simulink model "lss_online"  (R2022b)
settings: Solver=FixedStepAuto  StartTime=0.0  StopTime=Inf  FixedStep=0.001  RelTol=1e-3  EnableMultiTasking=on
InitFcn:
  | clear mex
model workspace (MAT data in the model file):
  worldsim_instance : object (value not decoded)
values from neighbouring files (symbols this model uses):
  ADAS_Control_Mode = 1    [LSS_parameters.m]    (also in lss_ini_param.sldd = 1.0)
  AP_Transition_Rate = 0.5    [LSS_parameters.m]    (also in lss_ini_param.sldd = 0.8)
  butter_a = 1.0 -1.9911142922016536 0.99115359586893548    [lss_ini_param.sldd]
  butter_a_lka_out = 1.0 -1.5610180758007179 0.641351538057563    [lss_ini_param.sldd]
  butter_b = 9.825916820482009E-6 1.9651833640964018E-5 9.825916820482009E-6    [lss_ini_param.sldd]
  butter_b_lka_out = 0.020083365564211246 0.040166731128422492 0.020083365564211246    [lss_ini_param.sldd]
  index_variant_approaching_speed = 3.0    [lss_ini_param.sldd]
  LDW_Activity_Flag = 1    [LSS_parameters.m]    (also in lss_ini_param.sldd = 1.0)
  LDW_Freq_Hz = Sensor_Freq_worldsim    [LSS_parameters.m]    (also in lss_ini_param.sldd = 50.0)
  LDW_LaneGap_dydt_Warning = 50    [LSS_parameters.m]    (also in lss_ini_param.sldd = 50.0)
  LDW_LaneGap_Warning = [0.5 0.25]    [LSS_parameters.m]    (also in lss_ini_param.sldd = 0.5 0.25)
  LDW_Min_Speed = 60    [LSS_parameters.m]    (also in lss_ini_param.sldd = 60.0)
  LDW_Steer_Vibration_Amplitude = 5    [LSS_parameters.m]    (also in lss_ini_param.sldd = 5.0)
  LDW_Steer_Vibration_Freq = 25    [LSS_parameters.m]    (also in lss_ini_param.sldd = 25.0)
  LKA_Activity_Flag = 1    [LSS_parameters.m]    (also in lss_ini_param.sldd = 1.0)
  LKA_D = [0.2 0.3]    [LSS_parameters.m]    (also in lss_ini_param.sldd = 0.2 0.3)
  LKA_Dyn_Rate_Limiter_Gain = 0.1    [LSS_parameters.m]    (also in lss_ini_param.sldd)
  LKA_Dyn_Rate_Limiter_Power = 10    [LSS_parameters.m]    (also in lss_ini_param.sldd = 10.0)
  LKA_Error_dydt_Off = 1    [LSS_parameters.m]    (also in lss_ini_param.sldd = 1.0)
  LKA_Error_Max = 3    [LSS_parameters.m]    (also in lss_ini_param.sldd = 3.0)
  LKA_Error_Off = 0.5    [LSS_parameters.m]    (also in lss_ini_param.sldd)
  LKA_Freq_Hz = Sensor_Freq_worldsim    [LSS_parameters.m]    (also in lss_ini_param.sldd = 50.0)
  LKA_I = [0.025 0.05]    [LSS_parameters.m]    (also in lss_ini_param.sldd = 0.025 0.05)
  LKA_Lane_Gap_Activate = [0.25 0.125]    [LSS_parameters.m]    (also in lss_ini_param.sldd = -0.05 0.125)
  LKA_Lane_Gap_dydt_Activate = 50    [LSS_parameters.m]    (also in lss_ini_param.sldd = 50.0)
  LKA_Min_Speed = 60    [LSS_parameters.m]    (also in lss_ini_param.mat = 50; lss_ini_param.sldd = 50.0)
  LKA_On_Display_Freq = 5    [LSS_parameters.m]    (also in lss_ini_param.sldd = 5.0)
  LKA_P = [0.1 0.2]    [LSS_parameters.m]    (also in lss_ini_param.sldd = 0.1 0.2)
  LKA_Steer_Rate_Max_radps = 1    [LSS_parameters.m]    (also in lss_ini_param.sldd = 1.0)
  radar_source = 2    [LSS_parameters.m]    (also in lss_ini_param.sldd = 2.0)
  Sensor_Freq_worldsim = 50    [launcher.m]    (also in lss_ini_param.sldd = 50.0)
  target_speed = 72    [LSS_parameters.m]    (also in launcher.m = initCond.initialVelocity * 3.6)
  variant_approaching_speed = v_lat    [launcher.m]    (also in lss_ini_param.sldd = 0.2 0.3 0.4 0.5 0.6)
  vehicle_width = 1.86    [LSS_parameters.m]    (also in lss_ini_param.sldd = 2.05)
libraries: simulink x41, simwbSfunlib x40, slpidlib x3, viworldsim_lib x3
(part 2 of 2)

== system lss_online/INPUT/simple_cruise_control ==
  note: This is used to mantaint the target speed until controller action
  Cast To Double : DataTypeConversion  OutDataTypeStr=double  SaturateOnIntegerOverflow=off  RndMeth=Floor
  Compare To Constant4 : simulink/Logic and Bit Operations/Compare To Constant  relop===  const=0  OutDataTypeStr=boolean
  Compare To Constant5 : simulink/Logic and Bit Operations/Compare To Constant  relop===  const=0  OutDataTypeStr=boolean
  Constant : Constant  Value=0
  PID Controller : slpidlib/PID Controller  Controller=PI  Form=Parallel  TimeDomain=Discrete-time  UseExternalTs=off  SampleTime=-1  IntegratorMethod=Forward Euler  FilterMethod=Forward Euler  ControllerParametersSource=internal  P=40  I=10  UseKiTs=off  D=0  N=100  UseFilter=on  TunerSelectOption=Transfer Function Based (PID Tuner App)  InitialConditionSource=internal  InitialConditionForIntegrator=0  InitialConditionForFilter=0  DifferentiatorICPrevScaledInput=0  ExternalReset=none  TrackingMode=off  Kt=1  LimitOutput=on  SatLimitsSource=internal  UpperSaturationLimit=100  LowerSaturationLimit=0  LinearizeAsGain=on  AntiWindupMode=none  Kb=1  LimitIntegrator=off  UpperIntegratorSaturationLimit=inf  LowerIntegratorSaturationLimit=-inf  POutMin=[]  POutMax=[]  IOutMin=[]  IOutMax=[]  DOutMin=[]  DOutMax=[]  NOutMin=[]  NOutMax=[]  SumOutMin=[]  SumOutMax=[]  SaturationOutMin=[]  SaturationOutMax=[]  PParamMin=[]  PParamMax=[]  IParamMin=[]  IParamMax=[]  DParamMin=[]  DParamMax=[]  NParamMin=[]  NParamMax=[]  KbParamMin=[]  KbParamMax=[]  KtParamMin=[]  KtParamMax=[]  KbOutMin=[]  KbOutMax=[]  KtOutMin=[]  KtOutMax=[]  IntegratorOutMin=[]  IntegratorOutMax=[]  FilterOutMin=[]  FilterOutMax=[]  SumI1OutMin=[]  SumI1OutMax=[]  SumI2OutMin=[]  SumI2OutMax=[]  SumI3OutMin=[]  SumI3OutMax=[]  SumI4OutMin=[]  SumI4OutMax=[]  SumDOutMin=[]  SumDOutMax=[]  DifferentiatorOutMin=[]  DifferentiatorOutMax=[]  FilterDiffOutCoefMin=[]  FilterDiffOutCoefMax=[]  ReciprocalOutMin=[]  ReciprocalOutMax=[]  SumDenOutMin=[]  SumDenOutMax=[]  SumNumOutMin=[]  SumNumOutMax=[]  DivideOutMin=[]  DivideOutMax=[]  UdiffTsProdOutMin=[]  UdiffTsProdOutMax=[]  NTsProdOutMin=[]  NTsProdOutMax=[]  UintegralTsProdOutMin=[]  UintegralTsProdOutMax=[]  UngainTsProdOutMin=[]  UngainTsProdOutMax=[]  ClampingZeroOutDataTypeStr=Inherit: Inherit via back propagation  ClampingZeroOutMin=[]  ClampingZeroOutMax=[]  FilterDenConstantOutDataTypeStr=Inherit: Inherit via back propagation  FilterDenConstantOutMin=[]  FilterDenConstantOutMax=[]  PCopyOutDataTypeStr=Inherit: Inherit via back propagation  PCopyOutMin=[]  PCopyOutMax=[]  NCopyOutDataTypeStr=Inherit: Inherit via back propagation  NCopyOutMin=[]  NCopyOutMax=[]  IntegratorContinuousStateAttributes=''  IntegratorStateMustResolveToSignalObject=off  IntegratorRTWStateStorageClass=Auto  FilterContinuousStateAttributes=''  FilterStateMustResolveToSignalObject=off  FilterRTWStateStorageClass=Auto  ParallelPVariant=InternalParameters  IdealPVariant=Disabled  IVariant=InternalParameters  DVariant=Disabled  IntegratorVariant=Discrete  SatVariant=Enabled  AWVariant=Passthrough  PCopyVariant=Disabled  TRVariant=Disabled  FdbkBlocksVariant=Forward  IdealPFdbkVariant=Disabled  SatFdbkVariant=Disabled  DerivativeFilterVariant=Disabled  NVariant=Disabled  NCopyVariant=Disabled_SignalSpec  FilterICVariant=Disabled  IntegratorICVariant=InternalICs  ExternalResetVariant=Disabled  TRSumVariant=Passthrough  SumFdbkVariant=Disabled  SumVariant=Sum_PI  TsampFilterVariant=InternalTs  TsampNgainVariant=Passthrough  TsampIntegralVariant=Passthrough  ExternalSaturationOutDataTypeStr=Inherit: Same as second input
  Product : Product
  Sum : Sum  Inputs=+-
  target_speed_ : Constant  Value=target_speed
  tag scope: CC_clutch_demand=global, CC_throttle_demand=global
  wires:
  target_speed_/1 -> Sum/1
  Sum/1 -> PID Controller/1
  [Vehicle_Speed] -> Sum/2
  PID Controller/1 -> Product/1  "throttle"
  Product/1 -> Compare To Constant4/1, [CC_throttle_demand]
  Compare To Constant5/1 -> Product/2
  [AEB_Output_Brake] -> Compare To Constant5/1
  Compare To Constant4/1 -> Cast To Double/1
  Cast To Double/1 -> [CC_clutch_demand]
  Constant/1 -> [AEB_Output_Brake]

== system lss_online/LDW/LDW_LaneGap_Warning1 ==
  In1 : Inport
  ADAS_Control_Mode : Constant  Value=ADAS_Control_Mode
  LDW_LaneGap_Warning : Constant  Value=LDW_LaneGap_Warning(1)
  LDW_LaneGap_Warning1 : Constant  Value=LDW_LaneGap_Warning(2)  VectorParams1D=off
  Multiport Switch : MultiPortSwitch  Inputs=2  DataPortForDefault=Additional data port  DiagnosticForDefault=None  SaturateOnIntegerOverflow=off  InputSameDT=off
  Relational Operator : RelationalOperator  Operator=<  OutDataTypeStr=boolean  InputSameDT=off
  Out1 : Outport  VectorParamsAs1DForOutWhenUnconnected=off
  wires:
  ADAS_Control_Mode/1 -> Multiport Switch/1
  Multiport Switch/1 -> Relational Operator/2
  Relational Operator/1 -> Out1/1
  In1/1 -> Relational Operator/1
  LDW_LaneGap_Warning/1 -> Multiport Switch/4, Multiport Switch/2
  LDW_LaneGap_Warning1/1 -> Multiport Switch/3

== system lss_online/LKA/Discrete PID Controller ==
  In1 : Inport
  In2 : Inport  Port=2
  ADAS_Control_Mode : Constant  Value=ADAS_Control_Mode
  Demux : Demux  Outputs=3
  Discrete PID Controller : slpidlib/PID Controller  Controller=PID  Form=Parallel  TimeDomain=Discrete-time  UseExternalTs=off  SampleTime=1/LKA_Freq_Hz  IntegratorMethod=Forward Euler  FilterMethod=Forward Euler  ControllerParametersSource=external  P=LKA_P  I=LKA_I  UseKiTs=off  D=LKA_D  N=100  UseFilter=off  TunerSelectOption=Transfer Function Based (PID Tuner App)  InitialConditionSource=internal  InitialConditionForIntegrator=0  InitialConditionForFilter=0  DifferentiatorICPrevScaledInput=0  ExternalReset=either  TrackingMode=off  Kt=1  LimitOutput=off  SatLimitsSource=internal  UpperSaturationLimit=inf  LowerSaturationLimit=-inf  LinearizeAsGain=off  AntiWindupMode=clamping  Kb=1  LimitIntegrator=off  UpperIntegratorSaturationLimit=inf  LowerIntegratorSaturationLimit=-inf  POutMin=[]  POutMax=[]  IOutMin=[]  IOutMax=[]  DOutMin=[]  DOutMax=[]  NOutMin=[]  NOutMax=[]  SumOutMin=[]  SumOutMax=[]  SaturationOutMin=[]  SaturationOutMax=[]  PParamMin=[]  PParamMax=[]  IParamMin=[]  IParamMax=[]  DParamMin=[]  DParamMax=[]  NParamMin=[]  NParamMax=[]  KbParamMin=[]  KbParamMax=[]  KtParamMin=[]  KtParamMax=[]  KbOutMin=[]  KbOutMax=[]  KtOutMin=[]  KtOutMax=[]  IntegratorOutMin=[]  IntegratorOutMax=[]  FilterOutMin=[]  FilterOutMax=[]  SumI1OutMin=[]  SumI1OutMax=[]  SumI2OutMin=[]  SumI2OutMax=[]  SumI3OutMin=[]  SumI3OutMax=[]  SumI4OutMin=[]  SumI4OutMax=[]  SumDOutMin=[]  SumDOutMax=[]  DifferentiatorOutMin=[]  DifferentiatorOutMax=[]  FilterDiffOutCoefMin=[]  FilterDiffOutCoefMax=[]  ReciprocalOutMin=[]  ReciprocalOutMax=[]  SumDenOutMin=[]  SumDenOutMax=[]  SumNumOutMin=[]  SumNumOutMax=[]  DivideOutMin=[]  DivideOutMax=[]  UdiffTsProdOutMin=[]  UdiffTsProdOutMax=[]  NTsProdOutMin=[]  NTsProdOutMax=[]  UintegralTsProdOutMin=[]  UintegralTsProdOutMax=[]  UngainTsProdOutMin=[]  UngainTsProdOutMax=[]  ClampingZeroOutDataTypeStr=Inherit: Inherit via back propagation  ClampingZeroOutMin=[]  ClampingZeroOutMax=[]  FilterDenConstantOutDataTypeStr=Inherit: Inherit via back propagation  FilterDenConstantOutMin=[]  FilterDenConstantOutMax=[]  PCopyOutDataTypeStr=Inherit: Inherit via back propagation  PCopyOutMin=[]  PCopyOutMax=[]  NCopyOutDataTypeStr=Inherit: Inherit via back propagation  NCopyOutMin=[]  NCopyOutMax=[]  IntegratorContinuousStateAttributes=''  IntegratorStateMustResolveToSignalObject=off  IntegratorRTWStateStorageClass=Auto  FilterContinuousStateAttributes=''  FilterStateMustResolveToSignalObject=off  FilterRTWStateStorageClass=Auto  ParallelPVariant=ExternalParameters  IdealPVariant=Disabled  IVariant=ExternalParameters  DVariant=ExternalParameters  IntegratorVariant=Discrete  SatVariant=Disabled  AWVariant=Passthrough  PCopyVariant=Disabled  TRVariant=Disabled  FdbkBlocksVariant=Forward  IdealPFdbkVariant=Disabled  SatFdbkVariant=Disabled  DerivativeFilterVariant=Differentiator  NVariant=Passthrough  NCopyVariant=Disabled_SignalSpec  FilterICVariant=InternalICsDifferentiator  IntegratorICVariant=InternalICs  ExternalResetVariant=ExternalReset  TRSumVariant=Passthrough  SumFdbkVariant=Disabled  SumVariant=Sum_PID  TsampFilterVariant=InternalTs  TsampNgainVariant=Passthrough  TsampIntegralVariant=Passthrough  ExternalSaturationOutDataTypeStr=Inherit: Same as second input
  LKA_D(1) : Constant  Value=LKA_D(1)
  LKA_D(1)1 : Constant  Value=LKA_D(2)
  LKA_I(1) : Constant  Value=LKA_I(1)
  LKA_I(1)1 : Constant  Value=LKA_I(2)
  LKA_P(1) : Constant  Value=LKA_P(1)
  LKA_P(1)1 : Constant  Value=LKA_P(2)
  Multiport Switch : MultiPortSwitch  Inputs=2  DataPortForDefault=Additional data port  DiagnosticForDefault=None  SaturateOnIntegerOverflow=off  InputSameDT=off
  Mux : Mux  Inputs=3
  Mux1 : Mux  Inputs=3
  Out1 : Outport  VectorParamsAs1DForOutWhenUnconnected=off
  wires:
  In1/1 -> Discrete PID Controller/1
  In2/1 -> Discrete PID Controller/5
  Discrete PID Controller/1 -> Out1/1
  LKA_P(1)/1 -> Mux/1
  ADAS_Control_Mode/1 -> Multiport Switch/1
  Demux/2 -> Discrete PID Controller/3
  Demux/3 -> Discrete PID Controller/4
  Demux/1 -> Discrete PID Controller/2
  Mux1/1 -> Multiport Switch/3
  Mux/1 -> Multiport Switch/4, Multiport Switch/2
  LKA_I(1)/1 -> Mux/2
  LKA_D(1)/1 -> Mux/3
  LKA_P(1)1/1 -> Mux1/1
  LKA_I(1)1/1 -> Mux1/2
  LKA_D(1)1/1 -> Mux1/3
  Multiport Switch/1 -> Demux/1

== system lss_online/LKA/LKA_Lane_Gap_Activate ==
  In1 : Inport
  ADAS_Control_Mode : Constant  Value=ADAS_Control_Mode
  LKA_Lane_Gap_Activate : Constant  Value=LKA_Lane_Gap_Activate(1)
  LKA_Lane_Gap_Activate2 : Constant  Value=LKA_Lane_Gap_Activate(2)  VectorParams1D=off
  Multiport Switch : MultiPortSwitch  Inputs=2  DataPortForDefault=Additional data port  DiagnosticForDefault=None  SaturateOnIntegerOverflow=off  InputSameDT=off
  Relational Operator : RelationalOperator  Operator=<  OutDataTypeStr=boolean  InputSameDT=off
  Out1 : Outport  VectorParamsAs1DForOutWhenUnconnected=off
  wires:
  ADAS_Control_Mode/1 -> Multiport Switch/1
  Multiport Switch/1 -> Relational Operator/2
  Relational Operator/1 -> Out1/1
  In1/1 -> Relational Operator/1
  LKA_Lane_Gap_Activate/1 -> Multiport Switch/4, Multiport Switch/2
  LKA_Lane_Gap_Activate2/1 -> Multiport Switch/3

== system lss_online/LKA/Subsystem ==
  Clock : Inport
  Input_Signal : Inport  Port=2
  Delay : Delay  DelayLength=1000/LKA_Freq_Hz  InitialCondition=-1/LKA_Freq_Hz
  Delay1 : Delay  DelayLength=1000/LKA_Freq_Hz
  Delay2 : Delay  DelayLength=1000/LKA_Freq_Hz
  Lookup Table Dynamic : simulink/Lookup Tables/Lookup Table Dynamic  LookUpMeth=Interpolation-Use End Values  OutDataType=fixdt('double')  OutScaling=[]  OutputDataTypeScalingMode=Specify via dialog  OutDataTypeStr=fixdt('double')  DoSatur=off
  Vector Concatenate : Concatenate
  Vector Concatenate1 : Concatenate
  Zero-Order Hold1 : ZeroOrderHold  SampleTime=1/LKA_Freq_Hz
  Zero-Order Hold2 : ZeroOrderHold  SampleTime=1/LKA_Freq_Hz
  Zero-Order Hold3 : ZeroOrderHold  SampleTime=1e-3
  Zero-Order Hold4 : ZeroOrderHold  SampleTime=1e-3
  1kHz_Interpolation : Outport  VectorParamsAs1DForOutWhenUnconnected=off
  wires:
  Input_Signal/1 -> Zero-Order Hold1/1
  Zero-Order Hold1/1 -> Zero-Order Hold4/1
  Zero-Order Hold3/1 -> Delay/1, Vector Concatenate/2
  Zero-Order Hold2/1 -> Zero-Order Hold3/1
  Delay/1 -> Vector Concatenate/1
  Delay1/1 -> Lookup Table Dynamic/1
  Delay2/1 -> Vector Concatenate1/1
  Zero-Order Hold4/1 -> Delay2/1, Vector Concatenate1/2
  Vector Concatenate1/1 -> Lookup Table Dynamic/3
  Vector Concatenate/1 -> Lookup Table Dynamic/2
  Clock/1 -> Delay1/1, Zero-Order Hold2/1
  Lookup Table Dynamic/1 -> 1kHz_Interpolation/1

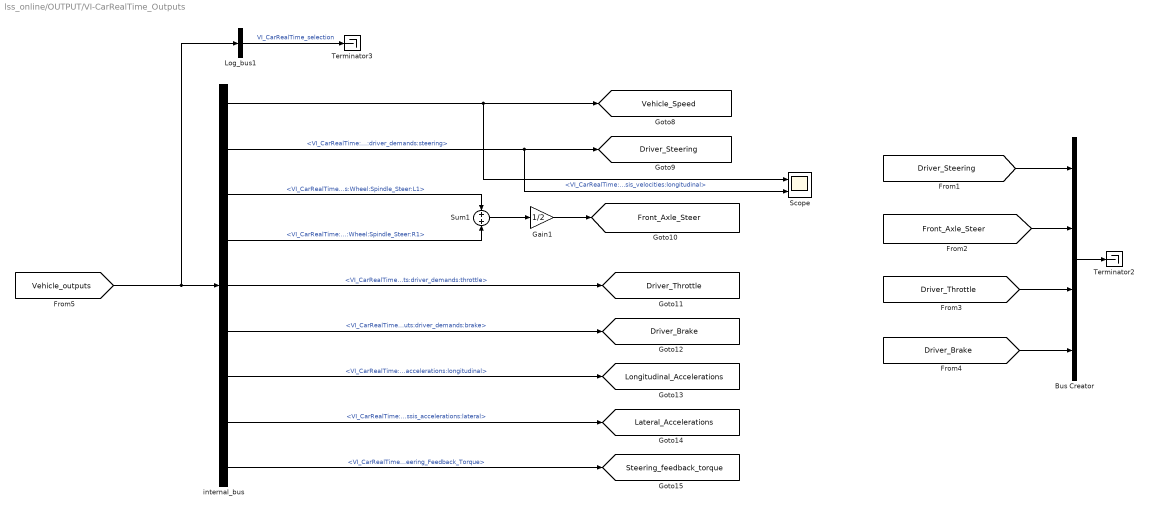
== system lss_online/OUTPUT/VI-CarRealTime_Outputs ==
  Bus Creator : BusCreator  Inputs=4
  Gain1 : Gain  Gain=1/2
  Log_bus1 : BusSelector  OutputSignals=VI_CarRealTime:Outputs:chassis_velocities:longitudinal,VI_CarRealTime:Outputs:driver_demands:steering,VI_CarRealTime:Outputs:Wheel:Spindle_Steer:L1,VI_CarRealTime:Outputs:Wheel:Spindle_Steer:R1,VI_CarRealTime:Outputs:driver_demands:throttle,VI_CarRealTime:Outputs:driver_demands:brake,VI_CarRealTime:Outputs:chassis_accelerations:longitudinal,VI_CarRealTime:Outputs:chassis_accelerations:lateral,VI_CarRealTime:Outputs:Steering_System:DriveSim_Steering_Feedback_Torque  OutputAsBus=on
  Scope : Scope  NumInputPorts=2
  Sum1 : Sum
  Terminator2 : Terminator
  Terminator3 : Terminator
  internal_bus : BusSelector  OutputSignals=VI_CarRealTime:Outputs:chassis_velocities:longitudinal,VI_CarRealTime:Outputs:driver_demands:steering,VI_CarRealTime:Outputs:Wheel:Spindle_Steer:L1,VI_CarRealTime:Outputs:Wheel:Spindle_Steer:R1,VI_CarRealTime:Outputs:driver_demands:throttle,VI_CarRealTime:Outputs:driver_demands:brake,VI_CarRealTime:Outputs:chassis_accelerations:longitudinal,VI_CarRealTime:Outputs:chassis_accelerations:lateral,VI_CarRealTime:Outputs:Steering_System:DriveSim_Steering_Feedback_Torque
  tag scope: Driver_Brake=global, Driver_Steering=global, Driver_Throttle=global, Front_Axle_Steer=global, Lateral_Accelerations=global, Longitudinal_Accelerations=global, Steering_feedback_torque=global, Vehicle_Speed=global
  wires:
  [Driver_Steering] -> Bus Creator/1
  [Front_Axle_Steer] -> Bus Creator/2
  [Driver_Throttle] -> Bus Creator/3
  [Driver_Brake] -> Bus Creator/4
  Bus Creator/1 -> Terminator2/1
  internal_bus/1 -> [Vehicle_Speed], Scope/1  "<VI_CarRealTime:Outputs:chassis_velocities:longitudinal>"
  Log_bus1/1 -> Terminator3/1  "VI_CarRealTime_selection"
  internal_bus/6 -> [Driver_Brake]  "<VI_CarRealTime:Outputs:driver_demands:brake>"
  internal_bus/3 -> Sum1/1  "<VI_CarRealTime:Outputs:Wheel:Spindle_Steer:L1>"
  internal_bus/7 -> [Longitudinal_Accelerations]  "<VI_CarRealTime:Outputs:chassis_accelerations:longitudinal>"
  [Vehicle_outputs] -> internal_bus/1, Log_bus1/1
  internal_bus/4 -> Sum1/2  "<VI_CarRealTime:Outputs:Wheel:Spindle_Steer:R1>"
  internal_bus/2 -> [Driver_Steering], Scope/2  "<VI_CarRealTime:Outputs:driver_demands:steering>"
  Gain1/1 -> [Front_Axle_Steer]
  internal_bus/8 -> [Lateral_Accelerations]  "<VI_CarRealTime:Outputs:chassis_accelerations:lateral>"
  internal_bus/5 -> [Driver_Throttle]  "<VI_CarRealTime:Outputs:driver_demands:throttle>"
  internal_bus/9 -> [Steering_feedback_torque]  "<VI_CarRealTime:Outputs:Steering_System:DriveSim_Steering_Feedback_Torque>"
  Sum1/1 -> Gain1/1

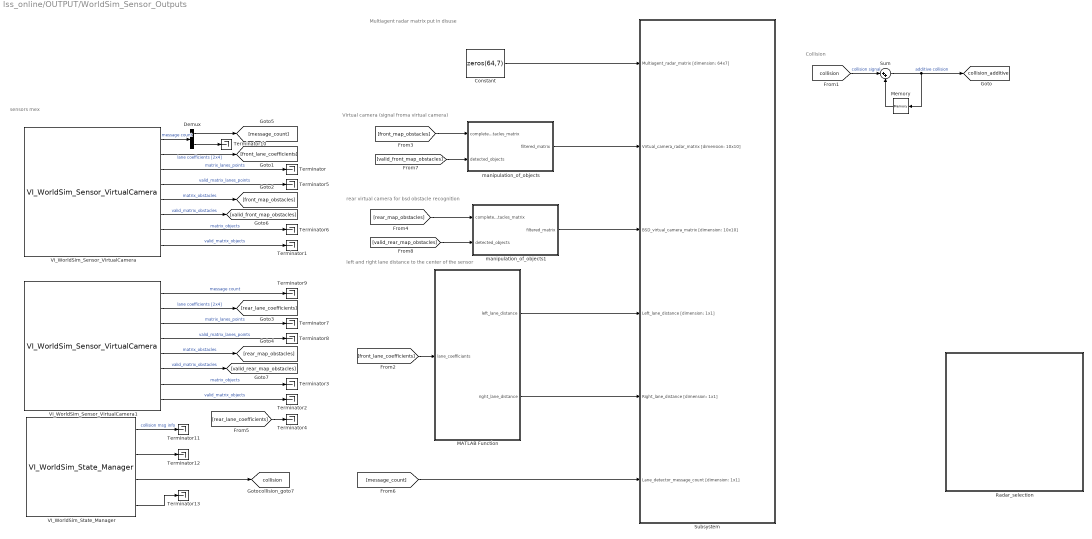
== system lss_online/OUTPUT/WorldSim_Sensor_Outputs ==
  note: Collision
  note: left and right lane distance to the center of the sensor
  note: Virtual camera (signal froma virtual camera)
  note: Multiagent radar matrix
      | put in disuse
  note: rear virtual camera for bsd obstacle recognition
  note: sensors mex
  Constant : Constant  Value=zeros(64,7)
  Demux : Demux  Outputs=2
  MATLAB Function : MATLAB Function  TreatAsAtomicUnit=on
  Memory : Memory  InheritSampleTime=on
  Radar_selection : Subsystem
  Subsystem : Subsystem
  Sum : Sum  Inputs=|++
  Terminator{,1..13} (14 alike) : Terminator
  VI_WorldSim_Sensor_VirtualCamera : viworldsim_lib/VI-WorldSim Sensors/VI_WorldSim_Sensor_VirtualCamera  worldsim_endpoint_ip=worldsim_instance.endpoint_ip  worldsim_endpoint_port=worldsim_instance.endpoint_port  worldsim_car_name='ego'  worldsim_sensor_name='Front_VirtualCam'  max_lanes=10  max_obstacles=10  worldsim_verbose=off
  VI_WorldSim_Sensor_VirtualCamera1 : viworldsim_lib/VI-WorldSim Sensors/VI_WorldSim_Sensor_VirtualCamera  worldsim_endpoint_ip=worldsim_instance.endpoint_ip  worldsim_endpoint_port=worldsim_instance.endpoint_port  worldsim_car_name='ego'  worldsim_sensor_name='Rear_VirtualCam'  max_lanes=10  max_obstacles=10  worldsim_verbose=off
  VI_WorldSim_State_Manager : viworldsim_lib/VI-WorldSim Sensors/VI_WorldSim_State_Manager  worldsim_endpoint_ip=worldsim_instance.endpoint_ip  worldsim_endpoint_port=worldsim_instance.endpoint_port  worldsim_car_name='ego'  worldsim_verbose=off
  manipulation_of_objects : MATLAB Function  TreatAsAtomicUnit=on
  manipulation_of_objects1 : MATLAB Function  TreatAsAtomicUnit=on
  tag scope: collision=global, collision_additive=global
  wires:
  Sum/1 -> Memory/1, [collision_additive]  "additive collision"
  [collision] -> Sum/1  "collision signal"
  Memory/1 -> Sum/2
  MATLAB Function/1(left_lane_distance) -> Subsystem/4(Left_lane_distance [dimension: 1x1])
  [message_count] -> Subsystem/6(Lane_detector_message_count [dimension: 1x1])
  manipulation_of_objects1/1(filtered_matrix) -> Subsystem/3(BSD_virtual_camera_matrix [dimension: 10x10])
  manipulation_of_objects/1(filtered_matrix) -> Subsystem/2(Virtual_camera_radar_matrix [dimension: 10x10])
  Constant/1 -> Subsystem/1(Multiagent_radar_matrix [dimension: 64x7])
  [valid_rear_map_obstacles] -> manipulation_of_objects1/2(detected_objects)
  MATLAB Function/2(right_lane_distance) -> Subsystem/5(Right_lane_distance [dimension: 1x1])
  [front_lane_coefficients] -> MATLAB Function/1(lane_coefficiants)
  [rear_map_obstacles] -> manipulation_of_objects1/1(complete_obstacles_matrix)
  [valid_front_map_obstacles] -> manipulation_of_objects/2(detected_objects)
  [front_map_obstacles] -> manipulation_of_objects/1(complete_obstacles_matrix)
  VI_WorldSim_Sensor_VirtualCamera/1 -> Demux/1  "message count"
  VI_WorldSim_State_Manager/1 -> Terminator11/1  "collision msg info"
  VI_WorldSim_Sensor_VirtualCamera/8 -> Terminator1/1  "valid_matrix_objects"
  VI_WorldSim_Sensor_VirtualCamera/5 -> [front_map_obstacles]  "matrix_obstacles"
  VI_WorldSim_Sensor_VirtualCamera/4 -> Terminator5/1  "valid_matrix_lanes_points"
  VI_WorldSim_Sensor_VirtualCamera/6 -> [valid_front_map_obstacles]  "valid_matrix_obstacles"
  VI_WorldSim_Sensor_VirtualCamera1/2 -> [rear_lane_coefficients]  "lane coefficients [2x4]"
  VI_WorldSim_Sensor_VirtualCamera/3 -> Terminator/1  "matrix_lanes_points"
  VI_WorldSim_Sensor_VirtualCamera1/1 -> Terminator9/1  "message count"
  VI_WorldSim_Sensor_VirtualCamera1/7 -> Terminator3/1  "matrix_objects"
  VI_WorldSim_Sensor_VirtualCamera1/8 -> Terminator2/1  "valid_matrix_objects"
  VI_WorldSim_Sensor_VirtualCamera/7 -> Terminator6/1  "matrix_objects"
  VI_WorldSim_Sensor_VirtualCamera/2 -> [front_lane_coefficients]  "lane coefficients [2x4]"
  VI_WorldSim_Sensor_VirtualCamera1/4 -> Terminator8/1  "valid_matrix_lanes_points"
  VI_WorldSim_State_Manager/3 -> [collision]
  VI_WorldSim_Sensor_VirtualCamera1/3 -> Terminator7/1  "matrix_lanes_points"
  [rear_lane_coefficients] -> Terminator4/1
  Demux/2 -> Terminator10/1
  VI_WorldSim_Sensor_VirtualCamera1/5 -> [rear_map_obstacles]  "matrix_obstacles"
  VI_WorldSim_Sensor_VirtualCamera1/6 -> [valid_rear_map_obstacles]  "valid_matrix_obstacles"
  Demux/1 -> [message_count]
  VI_WorldSim_State_Manager/2 -> Terminator12/1
  VI_WorldSim_State_Manager/4 -> Terminator13/1

== system lss_online/OUTPUT/rough data reporting ==
  Cast To Double : DataTypeConversion  OutDataTypeStr=double  SaturateOnIntegerOverflow=off  RndMeth=Floor
  Cast To Double1 : DataTypeConversion  OutDataTypeStr=double  SaturateOnIntegerOverflow=off  RndMeth=Floor
  Clock : Clock
  Compare To Constant : simulink/Logic and Bit Operations/Compare To Constant  relop=<=  const=0.0  OutDataTypeStr=boolean
  Compare To Constant1 : simulink/Logic and Bit Operations/Compare To Constant  relop=<=  const=0.0  OutDataTypeStr=boolean
  Compare To Constant2 : simulink/Logic and Bit Operations/Compare To Constant  relop=>  const=0.1  OutDataTypeStr=boolean
  Product : Product
  Scope LDW_Steering_Torque_in_out : Scope  NumInputPorts=2
  Sum1 : Sum
  To Workspace : ToWorkspace  VariableName=number_collision  SampleTime=-1
      settings: Save2DSignal=2-D array (concatenate along first dimension)
  To Workspace1 : ToWorkspace  VariableName=longitudinal_accelerations  SampleTime=-1
      settings: Save2DSignal=2-D array (concatenate along first dimension)
  To Workspace2 : ToWorkspace  VariableName=lateral_accelerations  SampleTime=-1
      settings: Save2DSignal=2-D array (concatenate along first dimension)
  To Workspace3 : ToWorkspace  VariableName=crossed_lanes  SampleTime=-1
      settings: Save2DSignal=2-D array (concatenate along first dimension)
  wires:
  Clock/1 -> Compare To Constant2/1
  Compare To Constant1/1 -> Cast To Double1/1
  [Lateral_Accelerations] -> To Workspace2/1
  [LaneGap_right_ws] -> Compare To Constant1/1
  Cast To Double/1 -> Sum1/1
  Compare To Constant2/1 -> Product/2
  [collision_additive] -> To Workspace/1
  Compare To Constant/1 -> Cast To Double/1
  [Longitudinal_Accelerations] -> To Workspace1/1
  [LaneGap_left_ws] -> Compare To Constant/1
  Product/1 -> To Workspace3/1
  Cast To Double1/1 -> Sum1/2
  Sum1/1 -> Product/1
  [Steering_feedback_torque] -> Scope LDW_Steering_Torque_in_out/2  "Output Steering Wheel Torque"
  [LDW_Steering_Torque] -> Scope LDW_Steering_Torque_in_out/1  "LDW Additional Steering Assist torque"

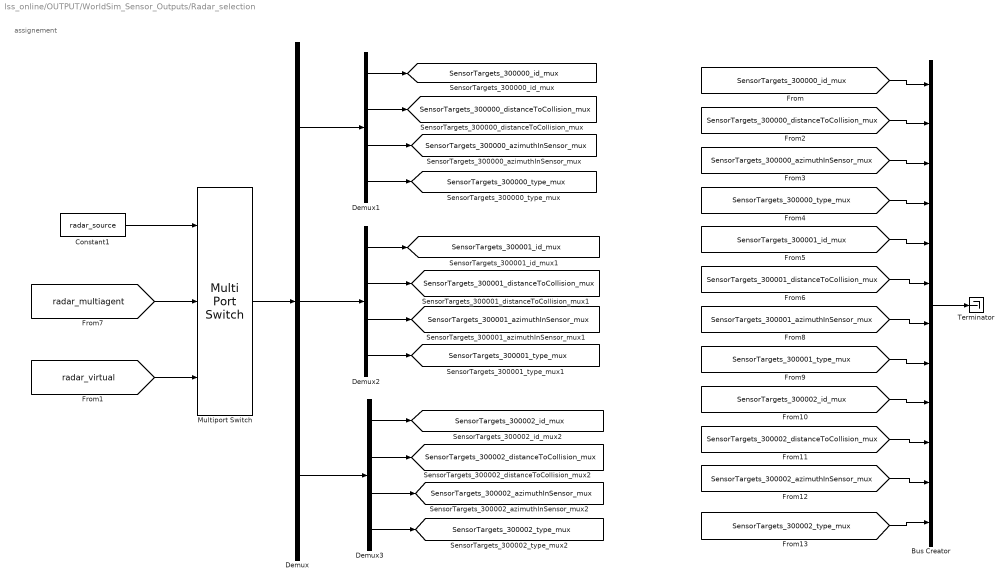
== system lss_online/OUTPUT/WorldSim_Sensor_Outputs/Radar_selection ==
  note: assignement
  Bus Creator : BusCreator  Inputs=12
  Constant1 : Constant  Value=radar_source
  Demux : Demux  Outputs=3
  Demux1 : Demux
  Demux2 : Demux
  Demux3 : Demux
  Multiport Switch : MultiPortSwitch  Inputs=2  SaturateOnIntegerOverflow=off  InputSameDT=off
  Terminator : Terminator
  tag scope: SensorTargets_300000_azimuthInSensor_mux=global, SensorTargets_300000_distanceToCollision_mux=global, SensorTargets_300000_id_mux=global, SensorTargets_300000_type_mux=global, SensorTargets_300001_azimuthInSensor_mux=global, SensorTargets_300001_distanceToCollision_mux=global, SensorTargets_300001_id_mux=global, SensorTargets_300001_type_mux=global, SensorTargets_300002_azimuthInSensor_mux=global, SensorTargets_300002_distanceToCollision_mux=global, SensorTargets_300002_id_mux=global, SensorTargets_300002_type_mux=global
  wires:
  [radar_virtual] -> Multiport Switch/3
  [radar_multiagent] -> Multiport Switch/2
  Constant1/1 -> Multiport Switch/1
  Multiport Switch/1 -> Demux/1
  Demux1/1 -> [SensorTargets_300000_id_mux]
  Demux3/4 -> [SensorTargets_300002_type_mux]
  Demux3/1 -> [SensorTargets_300002_id_mux]
  Demux1/4 -> [SensorTargets_300000_type_mux]
  Demux3/2 -> [SensorTargets_300002_distanceToCollision_mux]
  Demux2/3 -> [SensorTargets_300001_azimuthInSensor_mux]
  Demux1/2 -> [SensorTargets_300000_distanceToCollision_mux]
  Demux/1 -> Demux1/1
  Demux1/3 -> [SensorTargets_300000_azimuthInSensor_mux]
  Demux2/2 -> [SensorTargets_300001_distanceToCollision_mux]
  Demux3/3 -> [SensorTargets_300002_azimuthInSensor_mux]
  Demux2/4 -> [SensorTargets_300001_type_mux]
  Demux/3 -> Demux3/1
  Demux/2 -> Demux2/1
  Demux2/1 -> [SensorTargets_300001_id_mux]
  [SensorTargets_300000_id_mux] -> Bus Creator/1
  [SensorTargets_300000_distanceToCollision_mux] -> Bus Creator/2
  [SensorTargets_300000_azimuthInSensor_mux] -> Bus Creator/3
  [SensorTargets_300000_type_mux] -> Bus Creator/4
  [SensorTargets_300001_id_mux] -> Bus Creator/5
  [SensorTargets_300001_distanceToCollision_mux] -> Bus Creator/6
  [SensorTargets_300001_azimuthInSensor_mux] -> Bus Creator/7
  [SensorTargets_300001_type_mux] -> Bus Creator/8
  [SensorTargets_300002_id_mux] -> Bus Creator/9
  [SensorTargets_300002_distanceToCollision_mux] -> Bus Creator/10
  [SensorTargets_300002_azimuthInSensor_mux] -> Bus Creator/11
  [SensorTargets_300002_type_mux] -> Bus Creator/12
  Bus Creator/1 -> Terminator/1

== system lss_online/OUTPUT/WorldSim_Sensor_Outputs/Subsystem ==
  Multiagent_radar_matrix [dimension: 64x7] : Inport
  Virtual_camera_radar_matrix [dimension: 10x10] : Inport  Port=2
  BSD_virtual_camera_matrix [dimension: 10x10] : Inport  Port=3
  Left_lane_distance [dimension: 1x1] : Inport  Port=4
  Right_lane_distance [dimension: 1x1] : Inport  Port=5
  Lane_detector_message_count [dimension: 1x1] : Inport  Port=6
  Semitrack : Constant  Value=vehicle_width/2
  Terminator : Terminator
  Terminator1 : Terminator
  bsd setection from ostacle recognition : Subsystem
  lane marking acquisition : Subsystem
  "multiagent radar SimpleRadar_... are single double representing id, yaw, range, power_db, range_rate, yaw_rate, status" : Subsystem
  "obstacle detection " : Subsystem
  tag scope: frame_worldsim_left=global, frame_worldsim_right=global
  wires:
  Semitrack/1 -> lane marking acquisition/1(Semitrack), bsd setection from ostacle recognition/1(semitrack)
  Virtual_camera_radar_matrix [dimension: 10x10]/1 -> "obstacle detection "/1(Virtual_camera_obstacle_matrix)
  BSD_virtual_camera_matrix [dimension: 10x10]/1 -> bsd setection from ostacle recognition/2(BSD_matrix_obstalces)
  Left_lane_distance [dimension: 1x1]/1 -> lane marking acquisition/2(Left_lane_marking)
  Right_lane_distance [dimension: 1x1]/1 -> lane marking acquisition/3(Right_lane_marking)
  Multiagent_radar_matrix [dimension: 64x7]/1 -> "multiagent radar SimpleRadar_... are single double representing id, yaw, range, power_db, range_rate, yaw_rate, status"/1(Virtual_radar_obstacle_matrix)
  Lane_detector_message_count [dimension: 1x1]/1 -> [frame_worldsim_right], [frame_worldsim_left]
  [frame_worldsim_left] -> Terminator/1
  [frame_worldsim_right] -> Terminator1/1

== system lss_online/OUTPUT/WorldSim_Sensor_Outputs/Subsystem/bsd setection from ostacle recognition ==
  semitrack : Inport
  BSD_matrix_obstalces : Inport  Port=2
  Compare To Constant : simulink/Logic and Bit Operations/Compare To Constant  relop=>  const=30  OutDataTypeStr=boolean
  MATLAB Function3 : MATLAB Function  TreatAsAtomicUnit=on
  Product : Product
  Product1 : Product
  Terminator : Terminator
  Terminator1 : Terminator
  tag scope: BSD_left_ws=global, BSD_right_ws=global
  wires:
  Compare To Constant/1 -> Product1/1, Product/1
  BSD_matrix_obstalces/1 -> MATLAB Function3/1(u)
  Product/1 -> [BSD_left_ws]
  Product1/1 -> [BSD_right_ws]
  MATLAB Function3/2(right) -> Product1/2
  [Vehicle_Speed] -> Compare To Constant/1
  MATLAB Function3/1(left) -> Product/2
  semitrack/1 -> MATLAB Function3/2(semitrack)
  [BSD_left_ws] -> Terminator/1
  [BSD_right_ws] -> Terminator1/1

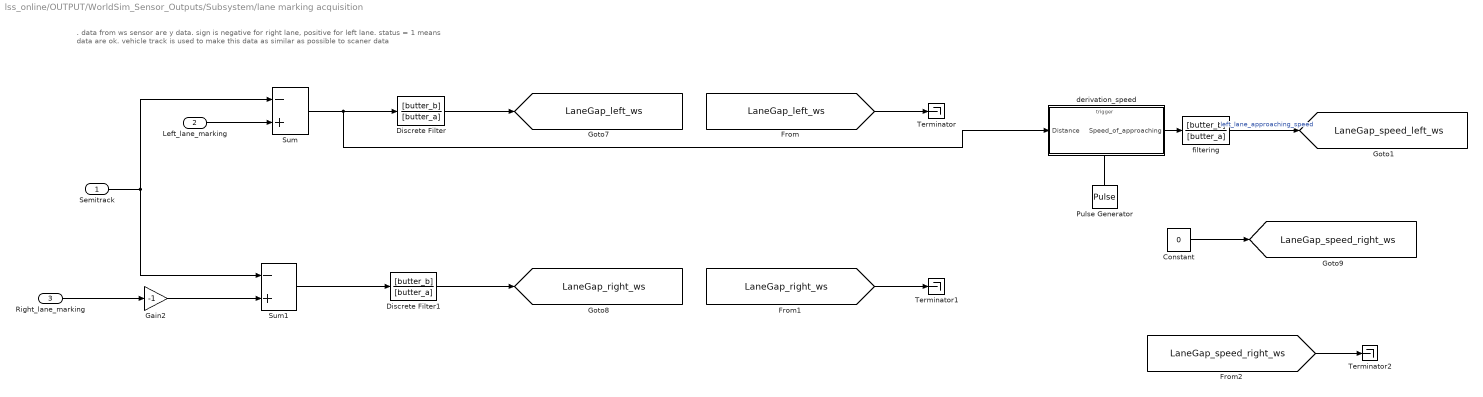
== system lss_online/OUTPUT/WorldSim_Sensor_Outputs/Subsystem/lane marking acquisition ==
  note: . data from ws sensor are y data. sign is negative for right lane, positive for left lane. status = 1 means data are ok. vehicle track is used to make this data as similar as possible to scaner data
  Semitrack : Inport
  Left_lane_marking : Inport  Port=2
  Right_lane_marking : Inport  Port=3
  Constant : Constant  Value=0
  Discrete Filter : DiscreteFilter  Numerator=[butter_b]  Denominator=[butter_a]  SampleTime=1e-3
  Discrete Filter1 : DiscreteFilter  Numerator=[butter_b]  Denominator=[butter_a]  SampleTime=1e-3
  Gain2 : Gain  Gain=-1
  Pulse Generator : DiscretePulseGenerator  PulseType=Time based  Period=1/Sensor_Freq_worldsim  PulseWidth=Sensor_Freq_worldsim*100/1000
  Sum : Sum  Inputs=-+
  Sum1 : Sum  Inputs=-+
  Terminator : Terminator
  Terminator1 : Terminator
  Terminator2 : Terminator
  derivation_speed : Subsystem
  filtering : DiscreteFilter  Numerator=[butter_b]  Denominator=[butter_a]  SampleTime=1e-3
  tag scope: LaneGap_left_ws=global, LaneGap_right_ws=global, LaneGap_speed_left_ws=global, LaneGap_speed_right_ws=global
  wires:
  Semitrack/1 -> Sum/1, Sum1/1
  Gain2/1 -> Sum1/2
  Sum/1 -> derivation_speed/1(Distance), Discrete Filter/1
  Left_lane_marking/1 -> Sum/2
  Sum1/1 -> Discrete Filter1/1
  Discrete Filter/1 -> [LaneGap_left_ws]
  Discrete Filter1/1 -> [LaneGap_right_ws]
  Right_lane_marking/1 -> Gain2/1
  [LaneGap_left_ws] -> Terminator/1
  [LaneGap_right_ws] -> Terminator1/1
  Pulse Generator/1 -> derivation_speed/Trigger
  derivation_speed/1(Speed_of_approaching) -> filtering/1
  filtering/1 -> [LaneGap_speed_left_ws]  "left_lane_approaching_speed"
  Constant/1 -> [LaneGap_speed_right_ws]
  [LaneGap_speed_right_ws] -> Terminator2/1

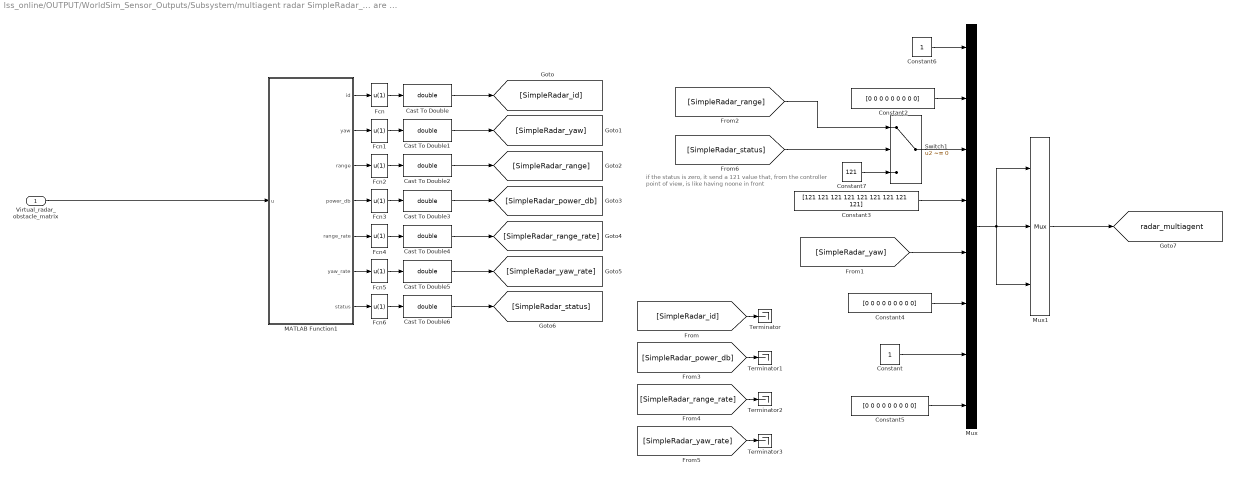
== system lss_online/OUTPUT/WorldSim_Sensor_Outputs/Subsystem/multiagent radar SimpleRadar_... are single double representing id, yaw, range, power_db, range_rate, yaw_rate, status ==
  note: if the status is zero, it send a 121 value that,
      | from the controller point of view, is like having noone in front
  Virtual_radar_obstacle_matrix : Inport
  Cast To Double{,1..6} (7 alike) : DataTypeConversion  OutDataTypeStr=double  SaturateOnIntegerOverflow=off  RndMeth=Floor
  Constant : Constant
  Constant2 : Constant  Value=[0 0 0 0 0 0 0 0 0]
  Constant3 : Constant  Value=[121 121 121 121 121 121 121 121 121]
  Constant4 : Constant  Value=[0 0 0 0 0 0 0 0 0]
  Constant5 : Constant  Value=[0 0 0 0 0 0 0 0 0]
  Constant6 : Constant
  Constant7 : Constant  Value=121
  Fcn{,1..6} (7 alike) : Fcn  Expr=u(1)
  MATLAB Function1 : MATLAB Function  TreatAsAtomicUnit=on
  Mux : Mux  Inputs=8
  Mux1 : Mux  Inputs=3
  Switch1 : Switch  Criteria=u2 ~= 0  SaturateOnIntegerOverflow=off  InputSameDT=off
  Terminator{,1..3} (4 alike) : Terminator
  tag scope: radar_multiagent=global
  wires:
  Virtual_radar_obstacle_matrix/1 -> MATLAB Function1/1(u)
  MATLAB Function1/6(yaw_rate) -> Fcn5/1
  Cast To Double3/1 -> [SimpleRadar_power_db]
  Cast To Double5/1 -> [SimpleRadar_yaw_rate]
  MATLAB Function1/1(id) -> Fcn/1
  Fcn4/1 -> Cast To Double4/1
  Cast To Double2/1 -> [SimpleRadar_range]
  Fcn5/1 -> Cast To Double5/1
  MATLAB Function1/2(yaw) -> Fcn1/1
  Cast To Double/1 -> [SimpleRadar_id]
  MATLAB Function1/7(status) -> Fcn6/1
  Fcn1/1 -> Cast To Double1/1
  Fcn6/1 -> Cast To Double6/1
  Fcn/1 -> Cast To Double/1
  Cast To Double4/1 -> [SimpleRadar_range_rate]
  MATLAB Function1/5(range_rate) -> Fcn4/1
  Cast To Double1/1 -> [SimpleRadar_yaw]
  MATLAB Function1/4(power_db) -> Fcn3/1
  Fcn2/1 -> Cast To Double2/1
  Fcn3/1 -> Cast To Double3/1
  MATLAB Function1/3(range) -> Fcn2/1
  Cast To Double6/1 -> [SimpleRadar_status]
  Switch1/1 -> Mux/3
  [SimpleRadar_yaw] -> Mux/5
  [SimpleRadar_status] -> Switch1/2
  Constant3/1 -> Mux/4
  Mux/1 -> Mux1/3, Mux1/1, Mux1/2
  Constant5/1 -> Mux/8
  Constant6/1 -> Mux/1
  Constant/1 -> Mux/7
  Constant4/1 -> Mux/6
  [SimpleRadar_yaw_rate] -> Terminator3/1
  Constant7/1 -> Switch1/3
  Constant2/1 -> Mux/2
  [SimpleRadar_range_rate] -> Terminator2/1
  [SimpleRadar_range] -> Switch1/1
  Mux1/1 -> [radar_multiagent]
  [SimpleRadar_id] -> Terminator/1
  [SimpleRadar_power_db] -> Terminator1/1

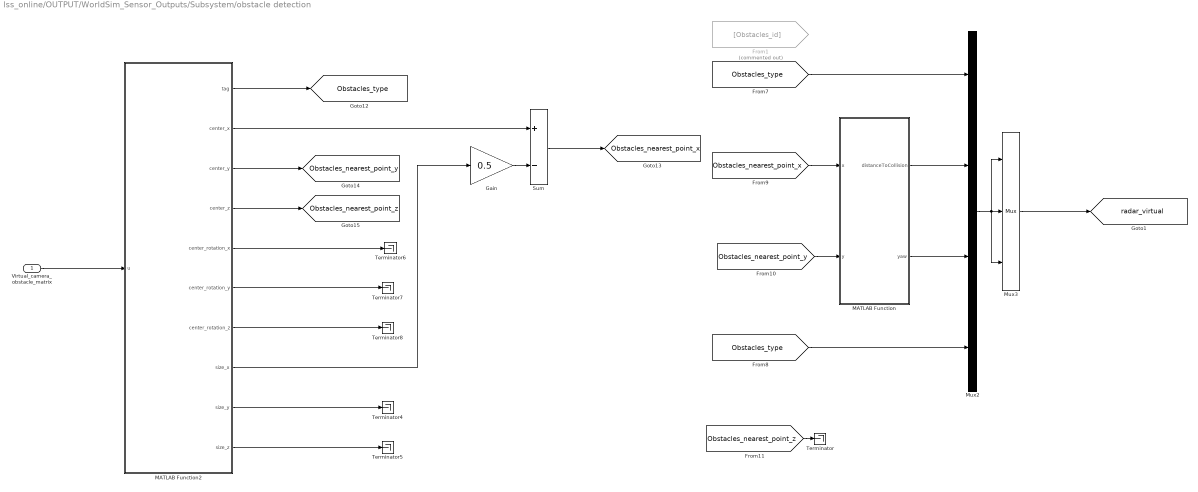
== system lss_online/OUTPUT/WorldSim_Sensor_Outputs/Subsystem/obstacle detection  ==
  Virtual_camera_obstacle_matrix : Inport
  From1 : From  Commented=on  GotoTag=Obstacles_id
  Gain : Gain  Gain=0.5
  MATLAB Function : MATLAB Function  TreatAsAtomicUnit=on
  MATLAB Function2 : MATLAB Function  TreatAsAtomicUnit=on
  Mux2 : Mux
  Mux3 : Mux  Inputs=3
  Sum : Sum  Inputs=+-
  Terminator{,4..8} (6 alike) : Terminator
  tag scope: Obstacles_nearest_point_x=global, Obstacles_nearest_point_y=global, Obstacles_nearest_point_z=global, Obstacles_type=global, radar_virtual=global
  wires:
  MATLAB Function2/1(tag) -> [Obstacles_type]
  Virtual_camera_obstacle_matrix/1 -> MATLAB Function2/1(u)
  Mux3/1 -> [radar_virtual]
  [Obstacles_nearest_point_x] -> MATLAB Function/1(x)
  [Obstacles_type] -> Mux2/4
  Mux2/1 -> Mux3/2, Mux3/1, Mux3/3
  [Obstacles_nearest_point_y] -> MATLAB Function/2(y)
  MATLAB Function/1(distanceToCollision) -> Mux2/2
  [Obstacles_type] -> Mux2/1
  [Obstacles_nearest_point_z] -> Terminator/1
  MATLAB Function/2(yaw) -> Mux2/3
  MATLAB Function2/3(center_y) -> [Obstacles_nearest_point_y]
  MATLAB Function2/4(center_z) -> [Obstacles_nearest_point_z]
  MATLAB Function2/5(center_rotation_x) -> Terminator6/1
  MATLAB Function2/6(center_rotation_y) -> Terminator7/1
  MATLAB Function2/7(center_rotation_z) -> Terminator8/1
  MATLAB Function2/9(size_y) -> Terminator4/1
  MATLAB Function2/10(size_z) -> Terminator5/1
  MATLAB Function2/8(size_x) -> Gain/1
  MATLAB Function2/2(center_x) -> Sum/1
  Gain/1 -> Sum/2
  Sum/1 -> [Obstacles_nearest_point_x]

== system lss_online/OUTPUT/WorldSim_Sensor_Outputs/Subsystem/lane marking acquisition/derivation_speed ==
  Distance : Inport
  Trigger : TriggerPort  VariantControl=Variant  PortDimensions=1
  Discrete Derivative : simulink/Discrete/Discrete Derivative  gainval=1.0  ICPrevScaledInput=0.0  OutMin=[]  OutMax=[]  OutDataType=fixdt(1, 16)  OutScaling=2^-10  DoSatur=off
  Gain : Gain  Gain=-1
  Speed_of_approaching : Outport
  wires:
  Discrete Derivative/1 -> Gain/1
  Gain/1 -> Speed_of_approaching/1
  Distance/1 -> Discrete Derivative/1

== matlab function lss_online/OUTPUT/WorldSim_Sensor_Outputs/manipulation_of_objects1 ==
  data: complete_obstacles_matrix input; filtered_matrix output; detected_objects input
function filtered_matrix = fcn(complete_obstacles_matrix, detected_objects)

% computations

filtered_matrix = complete_obstacles_matrix;

filtered_matrix(:,((detected_objects+1):size(filtered_matrix,2))) = 0;

== matlab function lss_online/LKA/MATLAB Function ==
  data: u input; y output
function y = fcn(u)

if u == 0
    y=1e-6;
else
    y=u;
end

end

== matlab function lss_online/OUTPUT/WorldSim_Sensor_Outputs/MATLAB Function ==
  data: lane_coefficiants input; left_lane_distance output; right_lane_distance output
function [left_lane_distance, right_lane_distance] = fcn(lane_coefficiants)

left_lane_distance = lane_coefficiants(1,1);
right_lane_distance = lane_coefficiants(2,1);

== matlab function lss_online/OUTPUT/WorldSim_Sensor_Outputs/manipulation_of_objects ==
  data: complete_obstacles_matrix input; filtered_matrix output; detected_objects input
function filtered_matrix = fcn(complete_obstacles_matrix, detected_objects)

% computations

filtered_matrix = complete_obstacles_matrix;

filtered_matrix(:,((detected_objects+1):size(filtered_matrix,2))) = 0;

== matlab function lss_online/OUTPUT/WorldSim_Sensor_Outputs/Subsystem/multiagent radar SimpleRadar_... are single double representing id, yaw, range, power_db, range_rate, yaw_rate, status/MATLAB Function1 ==
  data: u input; id output; yaw output; range output; power_db output; range_rate output; yaw_rate output; status output
function [id, yaw, range, power_db, range_rate, yaw_rate,status] = fcn(u)

id = u(:,1);
yaw = u(:,2);
range = u(:,3);
power_db = u(:,4);
range_rate = u(:,5);
yaw_rate = u(:,6);
status = u(:,7);

== matlab function lss_online/OUTPUT/WorldSim_Sensor_Outputs/Subsystem/obstacle detection /MATLAB Function2 ==
  data: u input; tag output; center_x output; center_y output; center_z output; center_rotation_x output; center_rotation_y output; center_rotation_z output; size_x output; size_y output; size_z output
function [tag, center_x, center_y, center_z, center_rotation_x, center_rotation_y, center_rotation_z, size_x, size_y, size_z] = fcn(u)

% this is the id tag that is assigned by ws at every scenario load
tag = (u(1,:))';
center_x = (u(2,:))';
center_y = (u(3,:))';
center_z = (u(4,:))';
center_rotation_x = (u(5,:))';
center_rotation_y = (u(6,:))';
center_rotation_z = (u(7,:))';
size_x = (u(8,:))';
size_y = (u(9,:))';
size_z = (u(10,:))';

%% identification of nearest box

% [index,index2]=min(u(:,3));
% 
% id = u(index,1);
% type = u(index,2);
% center_x = u(index,3);
% center_y = u(index,4);
% center_z = u(index,5);
% width = u(index,6);
% height = u(index,7);

== matlab function lss_online/OUTPUT/WorldSim_Sensor_Outputs/Subsystem/obstacle detection /MATLAB Function ==
  data: x input; distanceToCollision output; y input; yaw output
function [distanceToCollision, yaw] = fcn(x, y)

x(x==0)=121;
y(y==0)=121;

yaw = atan(y./x);
distanceToCollision=x./cos(yaw);
distanceToCollision(x==121)=121;

== matlab function lss_online/OUTPUT/WorldSim_Sensor_Outputs/Subsystem/bsd setection from ostacle recognition/MATLAB Function3 ==
  data: u input; semitrack input; left output; right output
function [left, right] = fcn(u, semitrack)
left=0;
right=0;

% [x,index] = min(nonzeros(u(:,3)));
x = (u(2,:))';
y = (u(3,:))';
% yaw = atan(y./x);
% distanceToCollision=x./cos(yaw);
index_left=find((y < -semitrack).*(y > -5),1);
index_right=find((y > semitrack).*(y < 5),1);
% .*(y > -3).*(x < 25)
if (~isempty(index_left))
    left = 1;
end
if (~isempty(index_right))
    right=1;
end
